simulink library "getFluidDynamicCenters_ul"  (R2018b)
settings: Solver=VariableStepAuto  StartTime=0.0  StopTime=10.0  RelTol=1e-3
settings Model: Creator=mcobb  LastModifiedBy=mcobb

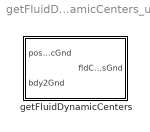
== system getFluidDynamicCenters_ul ==
  getFluidDynamicCenters : Subsystem  mask{vcl=0}
      mask prompts: vcl "Vehicle Object"

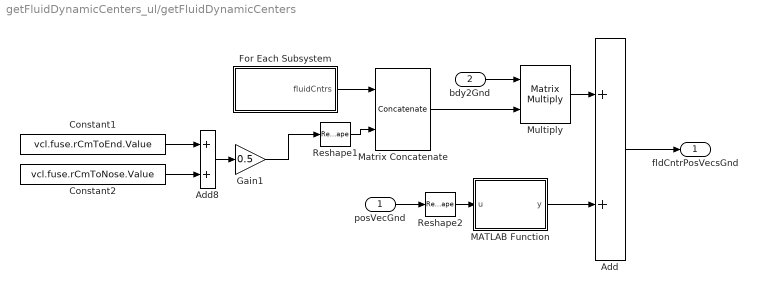
== system getFluidDynamicCenters_ul/getFluidDynamicCenters ==
  posVecGnd : Inport
  bdy2Gnd : Inport  Port=2
  Add : Sum
  Add8 : Sum
  Constant1 : Constant  Value=vcl.fuse.rCmToEnd.Value
  Constant2 : Constant  Value=vcl.fuse.rCmToNose.Value
  For Each Subsystem : Subsystem  TreatAsAtomicUnit=on  mask{aeroStruct=vcl.struct('OCT.aeroSurf')}
      mask prompts: aeroStruct "Aero Structure"
  Gain1 : Gain  Gain=0.5
  MATLAB Function : MATLAB Function  TreatAsAtomicUnit=on
  Matrix Concatenate : Concatenate  Mode=Multidimensional array  ConcatenateDimension=2
  Multiply : Product  Multiplication=Matrix(*)
  Reshape1 : Reshape  OutputDimensionality=Column vector (2-D)
  Reshape2 : Reshape  OutputDimensionality=Column vector (2-D)
  fldCntrPosVecsGnd : Outport
  wires:
  bdy2Gnd/1 -> Multiply/1
  posVecGnd/1 -> Reshape2/1
  Add/1 -> fldCntrPosVecsGnd/1
  Reshape2/1 -> MATLAB Function/1(u)
  For Each Subsystem/1(fluidCntrs) -> Matrix Concatenate/1
  Multiply/1 -> Add/1
  Gain1/1 -> Reshape1/1
  Constant2/1 -> Add8/2
  Add8/1 -> Gain1/1
  Constant1/1 -> Add8/1
  Reshape1/1 -> Matrix Concatenate/2
  Matrix Concatenate/1 -> Multiply/2
  MATLAB Function/1(y) -> Add/2

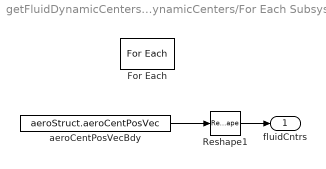
== system getFluidDynamicCenters_ul/getFluidDynamicCenters/For Each Subsystem ==
  For Each : ForEach  DisableCoverage=on  IterateSubsysMaskParameter=on  SubsysMaskParameterIterationDimension=2  IndexMode=One-based
  Reshape1 : Reshape  OutputDimensionality=Column vector (2-D)
  aeroCentPosVecBdy : Constant  Value=aeroStruct.aeroCentPosVec
  fluidCntrs : Outport  ConcatenationDimension=2
  wires:
  aeroCentPosVecBdy/1 -> Reshape1/1
  Reshape1/1 -> fluidCntrs/1

== matlab function getFluidDynamicCenters_ul/getFluidDynamicCenters/MATLAB Function ==
  data: u input; y output
function y = fcn(u)

y= repmat(u(:),[1 5]);
